simulink model "ame532Project1_GimbalDynamicsModel_2022b"  (R2022b)
settings: Solver=ode4  StartTime=0.0  StopTime=10  FixedStep=0.01  RelTol=1e-3
model workspace (MAT data in the model file):
  theta : Simulink.Parameter (value not decoded)
values from neighbouring files (symbols this model uses):
  a0_s2 = 0    [AeroData.m]
  a0_s3 = 0    [AeroData.m]
  a0_s4 = 0.05    [AeroData.m]
  a0_s5 = 0.05    [AeroData.m]
  CD0_s2 = 0.01    [AeroData.m]
  CD0_s3 = 0.01    [AeroData.m]
  CD0_s4 = 0.01    [AeroData.m]
  CD0_s5 = 0.01    [AeroData.m]
  CDa_s2 = 1    [AeroData.m]
  CDa_s3 = 1    [AeroData.m]
  CDa_s4 = 1    [AeroData.m]
  CDa_s5 = 1    [AeroData.m]
  CL0_s2 = 0    [AeroData.m]
  CL0_s3 = 0    [AeroData.m]
  CL0_s4 = 0.05    [AeroData.m]
  CL0_s5 = 0.05    [AeroData.m]
  CM0_s2 = 0    [AeroData.m]
  CM0_s3 = 0    [AeroData.m]
  CM0_s4 = -0.05    [AeroData.m]
  CM0_s5 = -0.05    [AeroData.m]
  CMa_s2 = 0    [AeroData.m]
  CMa_s3 = 0    [AeroData.m]
  CMa_s4 = 0    [AeroData.m]
  CMa_s5 = 0    [AeroData.m]
  e_s2 = 0.8    [AeroData.m]
  e_s3 = 0.8    [AeroData.m]
  e_s4 = 0.9    [AeroData.m]
  e_s5 = 0.9    [AeroData.m]
  i_s2 = 0    [AeroData.m]
  i_s3 = 0    [AeroData.m]
  i_s4 = 0.05    [AeroData.m]
  i_s5 = 0.05    [AeroData.m]
  Jxx = 1    [Sim_sixDOFdriverScript.m]
  Jxy = 0.    (= 0)    [Sim_sixDOFdriverScript.m]
  Jxz = 3    [Sim_sixDOFdriverScript.m]
  Jyx = 2    [Sim_sixDOFdriverScript.m]
  Jyy = 2    [Sim_sixDOFdriverScript.m]
  Jyz = 0    [Sim_sixDOFdriverScript.m]
  Jzx = Jxz    (= 3)    [Sim_sixDOFdriverScript.m]
  Jzy = Jyz    (= 0)    [Sim_sixDOFdriverScript.m]
  Jzz = 2    [Sim_sixDOFdriverScript.m]
  LL = 0.8    [Sim_sixDOFdriverScript.m]
  MM = 0.8    [Sim_sixDOFdriverScript.m]
  n_s2 = [0; 0; -1]    [AeroData.m]
  n_s3 = [0; 1; 0]    [AeroData.m]
  n_s4 = [0; 0; -1]    [AeroData.m]
  n_s5 = [0; 0; -1]    [AeroData.m]
  NN = 0.8    [Sim_sixDOFdriverScript.m]
  rEarth = 6378100    [Sim_sixDOFdriverScript.m]
  ro = 1.225    [AeroData.m]
undefined symbols (not defined in the file or in its folder): AR_s2, AR_s3, AR_s4, AR_s5, area_s2, area_s3, area_s4, area_s5, c_s2, c_s3, c_s4, c_s5, earthRadius, elevator_sA, leftaileron_sA, mixMatrixInv, rightaileron_sA, rudder_sA, totMass, x_S2_B_B, x_S3_B_B, x_S4_B_B, x_S5_B_B
libraries: simulink_extras x35, matrix_library x22, aerolibutil x8, aerolibfltsims x4, vrlib x4, aerolibtransform2 x2, sharedtransform x2, simulink x2, slpidlib x1, sharedutil x1
(part 4 of 5)

== matlab function ame532Project1_GimbalDynamicsModel_2022b/Gimbal Aircraft dynamic sim/aeroforce coefficient block/MATLAB Function3 ==
  data: alpha input; CM_0 input; CM_s output; CM_a input
function CM_s = calculate_CM_s(alpha,CM_0,CM_a)

CM_s = zeros(4,1);

for i = 1:4
    CM_s(i) = CM_0(i)+CM_a(i)*alpha(i);
end

== matlab function ame532Project1_GimbalDynamicsModel_2022b/Gimbal Aircraft dynamic sim/aeroforce & moment block/MATLAB Function ==
  data: CL_s input; Lift_s output; totalspeed input; area_s input
function Lift_s = calculate_Lift_s(CL_s,totalspeed,area_s)

Lift_s = zeros(4,1);
rho = 1.225; %kg/m3

for i = 1:4
    Lift_s(i) = CL_s(i)*0.5*rho*(totalspeed^2)*area_s(i);
end

end

== matlab function ame532Project1_GimbalDynamicsModel_2022b/Gimbal Aircraft dynamic sim/aeroforce & moment block/MATLAB Function1 ==
  data: aerosurface_matrix input; area_col output
function area_col = extract_area_col(aerosurface_matrix)

area_col = aerosurface_matrix(:,6);

end

== matlab function ame532Project1_GimbalDynamicsModel_2022b/IMU  Aircraft dynamic sim1/Rotational Kinematics/C_BN ==
  data: roll input; ZYXDCM output; pitch input; yaw input
function ZYXDCM = DCM_from_Euler(roll,pitch,yaw) % sequence is yaw pitch roll
    yaw_matrix = [cos(yaw) sin(yaw) 0;
                  -sin(yaw) cos(yaw) 0;
                  0 0 1];
    pitch_matrix = [cos(pitch) 0 -sin(pitch);
                    0           1           0;
                    sin(pitch) 0  cos(pitch)];
    roll_matrix = [1            0           0;
                    0          cos(roll)    sin(roll);
                    0           -sin(roll)  cos(roll)];
    ZYXDCM = roll_matrix*pitch_matrix*yaw_matrix;
end

== matlab function ame532Project1_GimbalDynamicsModel_2022b/Gimbal Aircraft dynamic sim/aeroforce & moment block/MATLAB Function2 ==
  data: CD_s input; Drag_s output; totalspeed input; area_s input
function Drag_s = calculate_Drag_s(CD_s,totalspeed,area_s)

Drag_s = zeros(4,1);
rho = 1.225; %kg/m3

for i = 1:4
    Drag_s(i) = CD_s(i)*0.5*rho*(totalspeed^2)*area_s(i);
end

end

== matlab function ame532Project1_GimbalDynamicsModel_2022b/Gimbal Aircraft dynamic sim/aeroforce & moment block/MATLAB Function3 ==
  data: CM_s input; Moment_s output; totalspeed input; area_s input; chord_s input
function Moment_s = calculate_Moment_s(CM_s,totalspeed,area_s,chord_s)

Moment_s = zeros(4,1);
rho = 1.225; %kg/m3

for i = 1:4
    Moment_s(i) = CM_s(i)*0.5*rho*(totalspeed^2)*area_s(i)*chord_s(i);
end

end

== matlab function ame532Project1_GimbalDynamicsModel_2022b/Gimbal Aircraft dynamic sim/aeroforce & moment block/MATLAB Function4 ==
  data: aerosurface_matrix input; chord_col output
function chord_col = extract_chord_col(aerosurface_matrix)

chord_col = aerosurface_matrix(:,4);

end

== matlab function ame532Project1_GimbalDynamicsModel_2022b/Gimbal Aircraft dynamic sim/aeroforce & moment block/MATLAB Function5 ==
  data: Lift_s input; F_w_s output; n_vector_s input; Drag_s input
function F_w_s = Calculate_F_w(Lift_s,n_vector_s,Drag_s)

F_w_s = zeros(3,4);

for i = 1:4
    F_w_s(:,i) = Lift_s(i).*n_vector_s(:,i) - [Drag_s(i) 0 0]';
end

== matlab function ame532Project1_GimbalDynamicsModel_2022b/Gimbal Aircraft dynamic sim/aeroforce & moment block/MATLAB Function6 ==
  data: n_vector_s input; M_s input; M_w_s output; F_b_s input; x_b_sb input
function M_w_s = Calculate_M_w(n_vector_s,M_s,F_b_s,x_b_sb)

M_w_s = zeros(3,4);

for i = 1:4
      M_w_s(:,i) = M_s(i)*[0 0 0; 0 0 -1; 0 1 0]*n_vector_s(:,i)+cross(x_b_sb(:,i),F_b_s(:,i));
%     M_w_s(:,i) = M_s(i)*[0 0 0; 0 0 -1; 0 1 0]*n_vector_s(:,i)+cross(F_b_s(:,i),x_b_sb(:,i));

end

== matlab function ame532Project1_GimbalDynamicsModel_2022b/Gimbal Aircraft dynamic sim/mass & aero property calculation/MATLAB Function1 ==
  data: aero_prop_matrix input; m_matrix input; x_b_s_ac output; cg_location input
function x_b_s_ac = calculate_x_b_sb(aero_prop_matrix,m_matrix,cg_location)
%this function calculates vector of each component to CM of aircraft

x_b_sb = zeros(3,4);
x_b_s_ac = zeros(3,4);
for i = 1:4
    x_b_s_ac(:,i) = m_matrix(i,5:7)' + [0.25*aero_prop_matrix(i,4) 0 0]';
    x_b_s_ac(:,i) = x_b_s_ac(:,i)- cg_location;

%     x_b_sb(:,i) = m_matrix(i,5:7)' - cg_location;

end

== matlab function ame532Project1_GimbalDynamicsModel_2022b/Gimbal Aircraft dynamic sim/aeroforce & moment block/MATLAB Function7 ==
  data: forcexyz_w_s_matrix input; force_xyz_w output
function force_xyz_w = sum_all_force_xyz(forcexyz_w_s_matrix)

force_xyz_w = zeros(3,1);

for i = 1:3
    force_xyz_w(i) = sum(forcexyz_w_s_matrix(i,:));
end

== matlab function ame532Project1_GimbalDynamicsModel_2022b/Gimbal Aircraft dynamic sim/aeroforce & moment block/MATLAB Function8 ==
  data: m_b_s input; moments_lmn_b output
function moments_lmn_b = sum_all_moments_b_s(m_b_s)

moments_lmn_b = zeros(3,1);

for i = 1:3
    moments_lmn_b(i) = sum(m_b_s(i,:));
end

== matlab function ame532Project1_GimbalDynamicsModel_2022b/Gimbal Aircraft dynamic sim/aeroforce & moment block/MATLAB Function9 ==
  data: DCM_WB output; v_body_ba input; alpha output; beta output; v_inf output
function [DCM_WB,alpha,beta,v_inf]  = construct_DCM_bw(v_body_ba)

alpha = atan2(v_body_ba(3),v_body_ba(1));
beta = asin(v_body_ba(2)/norm(v_body_ba));

DCM_WB = [cos(beta) sin(beta) 0; -sin(beta) cos(beta) 0; 0 0 1]*[cos(alpha) 0 sin(alpha); 0 1 0; -sin(alpha) 0 cos(alpha)];
v_inf = norm(v_body_ba);
end

== matlab function ame532Project1_GimbalDynamicsModel_2022b/IMU  Aircraft dynamic sim1/Rotational Kinematics/MATLAB Function3 ==
  data: p input; Cross_Product_Matrix output; q input; r input
function Cross_Product_Matrix = omega_to_cross_product_matrix(p,q,r)

    Cross_Product_Matrix =[0 -r q; r 0 -p; -q p 0];

end

== matlab function ame532Project1_GimbalDynamicsModel_2022b/IMU  Aircraft dynamic sim1/Rotational Kinematics/MATLAB Function4 ==
  data: DCM input; roll output; pitch output; yaw output
function [roll, pitch, yaw] = Euler_from_DCM(DCM)
   roll = atan2(DCM(2,3),DCM(3,3));
   pitch = -asin(DCM(1,3));
   yaw = atan2(DCM(1,2),DCM(1,1));
end

== matlab function ame532Project1_GimbalDynamicsModel_2022b/IMU  Aircraft dynamic sim1/Rotational Kinematics/C_EN1 ==
  data: roll input; ZYXDCM output; pitch input; yaw input
function ZYXDCM = DCM_from_Euler(roll,pitch,yaw) % sequence is yaw pitch roll
    yaw_matrix = [cos(yaw) sin(yaw) 0;
                  -sin(yaw) cos(yaw) 0;
                  0 0 1];
    pitch_matrix = [cos(pitch) 0 -sin(pitch);
                    0           1           0;
                    sin(pitch) 0  cos(pitch)];
    roll_matrix = [1            0           0;
                    0          cos(roll)    sin(roll);
                    0           -sin(roll)  cos(roll)];
    ZYXDCM = roll_matrix*pitch_matrix*yaw_matrix;
end

== matlab function ame532Project1_GimbalDynamicsModel_2022b/IMU  Aircraft dynamic sim1/Rotational Kinematics/MATLAB Function5 ==
  data: DCM input; roll output; pitch output; yaw output
function [roll, pitch, yaw] = Euler_from_DCM(DCM)
   roll = atan2(DCM(2,3),DCM(3,3));
   pitch = asin(DCM(1,3));
   yaw = atan2(DCM(1,2),DCM(1,1));
end

== matlab function ame532Project1_GimbalDynamicsModel_2022b/IMU  Aircraft dynamic sim1/Rotational Kinematics/MATLAB Function6 ==
  data: DCM input; roll output; pitch output; yaw output
function [roll, pitch, yaw] = Euler_from_DCM(DCM)
   roll = atan2(DCM(2,3),DCM(3,3));
   pitch = -asin(DCM(1,3));
   yaw = atan2(DCM(1,2),DCM(1,1));
end

== matlab function ame532Project1_GimbalDynamicsModel_2022b/IMU  Aircraft dynamic sim1/Rotational Kinematics/MATLAB Function7 ==
  data: quat input; roll output; pitch output; yaw output
function [roll, pitch, yaw] = Euler_from_Quat(quat)
    DCM = zeros(3,3);
    DCM(1) = (quat(1)^2+quat(2)^2-quat(3)^2-quat(4)^2);
    DCM(2) = 2*(quat(2)*quat(3)-quat(1)*quat(4));
    DCM(3) = 2*(quat(2)*quat(4)+quat(1)*quat(3));
    DCM(4) = 2*(quat(2)*quat(3)+quat(1)*quat(4));
    DCM(5) = (quat(1)^2-quat(2)^2+quat(3)^2-quat(4)^2);
    DCM(6) = 2*(quat(3)*quat(4)-quat(1)*quat(2));
    DCM(7) = 2*(quat(2)*quat(4)-quat(1)*quat(3));
    DCM(8) = 2*(quat(3)*quat(4)+quat(1)*quat(2));
    DCM(9) = (quat(1)^2-quat(2)^2-quat(3)^2+quat(4)^2);

    roll = atan2(DCM(2,3),DCM(3,3));
    pitch = -asin(DCM(1,3));
    yaw = atan2(DCM(1,2),DCM(1,1));
end

== matlab function ame532Project1_GimbalDynamicsModel_2022b/IMU  Aircraft dynamic sim1/Rotational Kinematics/MATLAB Function8 ==
  data: roll input; ZYXquat_inv output; pitch input; yaw input; ZYXquat output
function [ZYXquat_inv,ZYXquat] = Quat_from_Euler(roll,pitch,yaw)
    q_yaw = zeros(4,1);
    q_yaw(1) = cos(yaw/2);
    q_yaw(2:4,1) = sin(yaw/2)*[0 0 1]';

    q_pitch = zeros(4,1);
    q_pitch(1) = cos(pitch/2);
    q_pitch(2:4,1) = sin(pitch/2)*[0 1 0]';

    q_roll = zeros(4,1);
    q_roll(1) = cos(roll/2);
    q_roll(2:4,1) = sin(roll/2)*[1 0 0]';
    
    inv_q_yaw = [q_yaw(1);-q_yaw(2:4)];
    inv_q_pitch = [q_pitch(1);-q_pitch(2:4)];
    inv_q_roll = [q_roll(1);-q_roll(2:4)];

    ZYXquat_inv = quat_mult(quat_mult(inv_q_roll,inv_q_pitch),inv_q_yaw);
    ZYXquat = quat_mult(quat_mult(q_yaw,q_pitch),q_roll);

end

function quat = quat_mult(q1,q2)
    quat = zeros(4,1);
    quat(1) = q1(1)*q2(1)-q1(2)*q2(2)-q1(3)*q2(3)-q1(4)*q2(4);
    quat(2) = q1(1)*q2(2)+q1(2)*q2(1)+q1(3)*q2(4)-q1(4)*q2(3);
    quat(3) = q1(1)*q2(3)-q1(2)*q2(4)+q1(3)*q2(1)+q1(4)*q2(2);
    quat(4) = q1(1)*q2(4)+q1(2)*q2(3)-q1(3)*q2(2)+q1(4)*q2(1);
end

== matlab function ame532Project1_GimbalDynamicsModel_2022b/IMU  Aircraft dynamic sim1/Rotational Kinematics/MATLAB Function9 ==
  data: q1 input; quat output; q2 input
function quat = quat_mult(q1,q2)
    quat = zeros(4,1);
    quat(1) = q1(1)*q2(1)-q1(2)*q2(2)-q1(3)*q2(3)-q1(4)*q2(4);
    quat(2) = q1(1)*q2(2)+q1(2)*q2(1)+q1(3)*q2(4)-q1(4)*q2(3);
    quat(3) = q1(1)*q2(3)-q1(2)*q2(4)+q1(3)*q2(1)+q1(4)*q2(2);
    quat(4) = q1(1)*q2(4)+q1(2)*q2(3)-q1(3)*q2(2)+q1(4)*q2(1);
end

== matlab function ame532Project1_GimbalDynamicsModel_2022b/IMU  Aircraft dynamic sim1/Translational Kinematics/C_EN from LAX to ECEF ==
  data: lat input; ZYXDCM output; long input
function ZYXDCM = DCM_from_Euler(lat,long) % sequence of rotation is lat long
%     yaw_matrix = [cos(yaw) sin(yaw) 0;
%                   -sin(yaw) cos(yaw) 0;
%                   0 0 1];
    lat_matrix = [cos(lat) 0 -sin(lat);
                    0           1           0;
                    sin(lat) 0  cos(lat)];
    long_matrix = [1            0           0;
                    0          cos(-long)    sin(-long);
                    0           -sin(-long)  cos(-long)];

    adjust_matrix = [cos(pi/2) 0 -sin(pi/2);
                    0           1           0;
                    sin(pi/2) 0  cos(pi/2)];
    ZYXDCM = adjust_matrix*long_matrix*lat_matrix;
end

%this rotational matrix turns lat long coordinate into a new C_EN
%assuming the N CS is lat and longitudinally rotated, then you would do
%-longditudinal rotation then lat rotation, then rotate 90 degrees again to
%match ECEF

== matlab function ame532Project1_GimbalDynamicsModel_2022b/IMU  Aircraft dynamic sim1/Translational Kinematics/new C_EN base on cart. coordinate1 ==
  data: lat input; ZYXDCM output; long input
function ZYXDCM = DCM_from_Euler(lat,long) % sequence of rotation is lat long
%     yaw_matrix = [cos(yaw) sin(yaw) 0;
%                   -sin(yaw) cos(yaw) 0;
%                   0 0 1];
    lat_matrix = [cos(lat) 0 -sin(lat);
                    0           1           0;
                    sin(lat) 0  cos(lat)];
    long_matrix = [1            0           0;
                    0          cos(-long)    sin(-long);
                    0           -sin(-long)  cos(-long)];

    adjust_matrix = [cos(pi/2) 0 -sin(pi/2);
                    0           1           0;
                    sin(pi/2) 0  cos(pi/2)];
    ZYXDCM = adjust_matrix*long_matrix*lat_matrix;
end

%this rotational matrix turns lat long coordinate into a new C_EN
%assuming the N CS is lat and longitudinally rotated, then you would do
%-longditudinal rotation then lat rotation, then rotate 90 degrees again to
%match ECEF

== matlab function ame532Project1_GimbalDynamicsModel_2022b/IMU  Aircraft dynamic sim1/Unused tranlational kinmatics/C_EN4 ==
  data: roll input; ZYXDCM output; pitch input; yaw input
function ZYXDCM = DCM_from_Euler(roll,pitch,yaw) % sequence is yaw pitch roll
    yaw_matrix = [cos(yaw) sin(yaw) 0;
                  -sin(yaw) cos(yaw) 0;
                  0 0 1];
    pitch_matrix = [cos(pitch) 0 -sin(pitch);
                    0           1           0;
                    sin(pitch) 0  cos(pitch)];
    roll_matrix = [1            0           0;
                    0          cos(roll)    sin(roll);
                    0           -sin(roll)  cos(roll)];
    ZYXDCM = roll_matrix*pitch_matrix*yaw_matrix;
end

== matlab function ame532Project1_GimbalDynamicsModel_2022b/IMU  Aircraft dynamic sim1/aeroforce & moment block/MATLAB Function ==
  data: CL_s input; Lift_s output; totalspeed input; area_s input
function Lift_s = calculate_Lift_s(CL_s,totalspeed,area_s)

Lift_s = zeros(4,1);
rho = 1.225; %kg/m3

for i = 1:4
    Lift_s(i) = CL_s(i)*0.5*rho*(totalspeed^2)*area_s(i);
end

end

== matlab function ame532Project1_GimbalDynamicsModel_2022b/IMU  Aircraft dynamic sim1/aeroforce & moment block/MATLAB Function1 ==
  data: aerosurface_matrix input; area_col output
function area_col = extract_area_col(aerosurface_matrix)

area_col = aerosurface_matrix(:,6);

end

== matlab function ame532Project1_GimbalDynamicsModel_2022b/IMU  Aircraft dynamic sim1/Rotational Kinematics/C_EN2 ==
  data: roll input; ZYXDCM output; pitch input; yaw input
function ZYXDCM = DCM_from_Euler(roll,pitch,yaw) % sequence is yaw pitch roll
    yaw_matrix = [cos(yaw) -sin(yaw) 0;
                  sin(yaw) cos(yaw) 0;
                  0 0 1];
    pitch_matrix = [cos(pitch) 0 sin(pitch);
                    0           1           0;
                    -sin(pitch) 0  cos(pitch)];
    roll_matrix = [1            0           0;
                    0          cos(roll)    -sin(roll);
                    0           sin(roll)  cos(roll)];
    ZYXDCM = roll_matrix*pitch_matrix*yaw_matrix;
end

== matlab function ame532Project1_GimbalDynamicsModel_2022b/IMU  Aircraft dynamic sim1/aeroforce & moment block/MATLAB Function2 ==
  data: CD_s input; Drag_s output; totalspeed input; area_s input
function Drag_s = calculate_Drag_s(CD_s,totalspeed,area_s)

Drag_s = zeros(4,1);
rho = 1.225; %kg/m3

for i = 1:4
    Drag_s(i) = CD_s(i)*0.5*rho*(totalspeed^2)*area_s(i);
end

end

== matlab function ame532Project1_GimbalDynamicsModel_2022b/IMU  Aircraft dynamic sim1/aeroforce & moment block/MATLAB Function3 ==
  data: CM_s input; Moment_s output; totalspeed input; area_s input; chord_s input
function Moment_s = calculate_Moment_s(CM_s,totalspeed,area_s,chord_s)

Moment_s = zeros(4,1);
rho = 1.225; %kg/m3

for i = 1:4
    Moment_s(i) = CM_s(i)*0.5*rho*(totalspeed^2)*area_s(i)*chord_s(i);
end

end

== matlab function ame532Project1_GimbalDynamicsModel_2022b/IMU  Aircraft dynamic sim1/aeroforce & moment block/MATLAB Function4 ==
  data: aerosurface_matrix input; chord_col output
function chord_col = extract_chord_col(aerosurface_matrix)

chord_col = aerosurface_matrix(:,4);

end

== matlab function ame532Project1_GimbalDynamicsModel_2022b/IMU  Aircraft dynamic sim1/aeroforce & moment block/MATLAB Function5 ==
  data: Lift_s input; F_w_s output; n_vector_s input; Drag_s input
function F_w_s = Calculate_F_w(Lift_s,n_vector_s,Drag_s)

F_w_s = zeros(3,4);

for i = 1:4
    F_w_s(:,i) = Lift_s(i).*n_vector_s(:,i) - [Drag_s(i) 0 0]';
end

== matlab function ame532Project1_GimbalDynamicsModel_2022b/IMU  Aircraft dynamic sim1/aeroforce & moment block/MATLAB Function6 ==
  data: n_vector_s input; M_s input; M_w_s output; F_b_s input; x_b_sb input
function M_w_s = Calculate_M_w(n_vector_s,M_s,F_b_s,x_b_sb)

M_w_s = zeros(3,4);

for i = 1:4
      M_w_s(:,i) = M_s(i)*[0 0 0; 0 0 -1; 0 1 0]*n_vector_s(:,i)+cross(x_b_sb(:,i),F_b_s(:,i));
%     M_w_s(:,i) = M_s(i)*[0 0 0; 0 0 -1; 0 1 0]*n_vector_s(:,i)+cross(F_b_s(:,i),x_b_sb(:,i));

end

== matlab function ame532Project1_GimbalDynamicsModel_2022b/IMU  Aircraft dynamic sim1/aeroforce & moment block/MATLAB Function7 ==
  data: forcexyz_w_s_matrix input; force_xyz_w output
function force_xyz_w = sum_all_force_xyz(forcexyz_w_s_matrix)

force_xyz_w = zeros(3,1);

for i = 1:3
    force_xyz_w(i) = sum(forcexyz_w_s_matrix(i,:));
end

== matlab function ame532Project1_GimbalDynamicsModel_2022b/IMU  Aircraft dynamic sim1/aeroforce & moment block/MATLAB Function8 ==
  data: m_b_s input; moments_lmn_b output
function moments_lmn_b = sum_all_moments_b_s(m_b_s)

moments_lmn_b = zeros(3,1);

for i = 1:3
    moments_lmn_b(i) = sum(m_b_s(i,:));
end

== matlab function ame532Project1_GimbalDynamicsModel_2022b/IMU  Aircraft dynamic sim1/aeroforce & moment block/MATLAB Function9 ==
  data: DCM_WB output; v_body_ba input; alpha output; beta output; v_inf output
function [DCM_WB,alpha,beta,v_inf]  = construct_DCM_bw(v_body_ba)

alpha = atan2(v_body_ba(3),v_body_ba(1));
beta = asin(v_body_ba(2)/norm(v_body_ba));

DCM_WB = [cos(beta) sin(beta) 0; -sin(beta) cos(beta) 0; 0 0 1]*[cos(alpha) 0 sin(alpha); 0 1 0; -sin(alpha) 0 cos(alpha)];
v_inf = norm(v_body_ba);
end

== matlab function ame532Project1_GimbalDynamicsModel_2022b/IMU  Aircraft dynamic sim1/aeroforce coefficient block/MATLAB Function ==
  data: AR_matrix input; CL_a output
function CL_a = Calculate_CL_a(AR_matrix)

CL_a = zeros(4,1);

for i = 1:4
    CL_a(i) = 2*pi*(AR_matrix(i)/(2+AR_matrix(i)));
end

== matlab function ame532Project1_GimbalDynamicsModel_2022b/IMU  Aircraft dynamic sim1/aeroforce coefficient block/MATLAB Function1 ==
  data: CL0 input; CL_s output; CL_a input; alpha input
function CL_s = calculate_CL_s(CL0,CL_a,alpha)

CL_s = zeros(4,1);

for i = 1:4
    CL_s(i) = CL0(i)+CL_a(i)*alpha(i);
end

== matlab function ame532Project1_GimbalDynamicsModel_2022b/IMU  Aircraft dynamic sim1/aeroforce coefficient block/MATLAB Function2 ==
  data: CD_0 input; CD_a input; CD_s output; alpha_0 input; alpha input; CL_s input; e input; AR input
function CD_s = calculate_CD_s(CD_0,CD_a,alpha_0,alpha,CL_s,e,AR)
CD_s = zeros(4,1);

for i = 1:4
    
    CD_s(i) = CD_0(i) + CD_a(i)*(alpha(i)-alpha_0(i))^2+(CL_s(i)^2)/(pi*e(i)*AR(i));

end

== matlab function ame532Project1_GimbalDynamicsModel_2022b/IMU  Aircraft dynamic sim1/Rotational Kinematics/MATLAB Function2 ==
  data: phi input; H_matrix_inv output; theta input; psi input
function H_matrix_inv = inv_h_matrix_from_euler(phi,theta,psi)

H_matrix_inv = [1, tan(theta)*sin(phi), tan(theta)*cos(phi);
                0,      cos(phi),           -sin(phi);      
                0,     sin(phi)/cos(theta),   cos(phi)/cos(theta)];

end

== matlab function ame532Project1_GimbalDynamicsModel_2022b/IMU  Aircraft dynamic sim1/aeroforce coefficient block/MATLAB Function3 ==
  data: alpha input; CM_0 input; CM_s output; CM_a input
function CM_s = calculate_CM_s(alpha,CM_0,CM_a)

CM_s = zeros(4,1);

for i = 1:4
    CM_s(i) = CM_0(i)+CM_a(i)*alpha(i);
end

== matlab function ame532Project1_GimbalDynamicsModel_2022b/IMU  Aircraft dynamic sim1/aeroforce coefficient block/calculatie alpha ==
  data: i0 input; alpha output; v_B input; n_vector input; wind_w input; v_B_BA output; C_BN input
function [alpha,v_B_BA] = fcn(i0,v_B,n_vector,wind_w,C_BN)

alpha = zeros(4,1);
% this function calculates alpha that the aero surface sees

v_B_BA = v_B - C_BN*wind_w;

for i = 1:4
    alpha(i) = i0(i) - asin(dot(v_B_BA,n_vector(:,i))/norm(v_B_BA));
end

== matlab function ame532Project1_GimbalDynamicsModel_2022b/IMU  Aircraft dynamic sim1/aeroforce coefficient block/extract matrix function ==
  data: aero_surface_matrix input; AR_matrix output
function AR_matrix = Extract_AR(aero_surface_matrix)

AR_matrix = aero_surface_matrix(:,7);
end

== matlab function ame532Project1_GimbalDynamicsModel_2022b/IMU  Aircraft dynamic sim1/aeroforce coefficient block/extract matrix function1 ==
  data: aero_surface_matrix input; AR_matrix output
function AR_matrix = Extract_AR(aero_surface_matrix)

AR_matrix = aero_surface_matrix(:,7);
end

== matlab function ame532Project1_GimbalDynamicsModel_2022b/IMU  Aircraft dynamic sim1/mass & aero property calculation/CG calculation ==
  data: M_matrix input; cg_x output; cg_y output; cg_z output
function [cg_x, cg_y, cg_z] = CG_calc(M_matrix)

mass_col = M_matrix(:,1);
x_col = M_matrix(:,5);
y_col = M_matrix(:,6);
z_col = M_matrix(:,7);

cg_x = sum(mass_col.*x_col)/(sum(mass_col));
cg_y = sum(mass_col.*y_col)/(sum(mass_col));
cg_z = sum(mass_col.*z_col)/(sum(mass_col));

end

== matlab function ame532Project1_GimbalDynamicsModel_2022b/IMU  Aircraft dynamic sim1/mass & aero property calculation/MATLAB Function ==
  data: cg_location input; M_matrix input; J_matrix output
function J_matrix = fcn(cg_location,M_matrix)


mass_col = M_matrix(:,1);
x_dim = M_matrix(:,2);
y_dim = M_matrix(:,3);
z_dim = M_matrix(:,4);
x_loc = M_matrix(:,5);
y_loc = M_matrix(:,6);
z_loc = M_matrix(:,7);

Ixx = zeros(11,1);
Iyy = zeros(11,1);
Izz = zeros(11,1);
Ixz = zeros(11,1);
Izx = Ixz;
Ixy = zeros(11,1);
Iyx = Ixy;
Iyz = zeros(11,1);
Izy = Iyz;

J_matrix = zeros(3,3);

% all moment of inertial is calculated wrt to CG

for i = 1:11
    Ixx(i) = mass_col(i)*(y_dim(i)^2+z_dim(i)^2)/(12)+mass_col(i)*((y_loc(i)-cg_location(2))^2+(z_loc(i)-cg_location(3))^2); % check discussion post
    Iyy(i) = mass_col(i)*(x_dim(i)^2+z_dim(i)^2)/(12)+mass_col(i)*((x_loc(i)-cg_location(1))^2+(z_loc(i)-cg_location(3))^2);
    Izz(i) = mass_col(i)*(y_dim(i)^2+x_dim(i)^2)/(12)+mass_col(i)*((y_loc(i)-cg_location(2))^2+(x_loc(i)-cg_location(1))^2);
    Ixz(i) = mass_col(i)*((z_loc(i)-cg_location(3))*(x_loc(i)-cg_location(1)));
    Ixy(i) = mass_col(i)*((x_loc(i)-cg_location(1))*(y_loc(i)-cg_location(2)));
    Iyz(i) = mass_col(i)*((y_loc(i)-cg_location(2))*(z_loc(i)-cg_location(3)));


end

J_matrix(1,1) = sum(Ixx);
J_matrix(2,2) = sum(Iyy);
J_matrix(3,3) = sum(Izz);
J_matrix(1,2) = sum(Ixy);
J_matrix(2,1) = sum(Ixy);
J_matrix(1,3) = sum(Ixz);
J_matrix(3,1) = sum(Ixz);
J_matrix(2,3) = sum(Iyz);
J_matrix(3,2) = sum(Iyz);

J_matrix = J_matrix./1000;
end

== matlab function ame532Project1_GimbalDynamicsModel_2022b/IMU  Aircraft dynamic sim1/mass & aero property calculation/MATLAB Function1 ==
  data: aero_prop_matrix input; m_matrix input; x_b_s_ac output; cg_location input
function x_b_s_ac = calculate_x_b_sb(aero_prop_matrix,m_matrix,cg_location)
%this function calculates vector of each component to CM of aircraft

x_b_sb = zeros(3,4);
x_b_s_ac = zeros(3,4);
for i = 1:4
    x_b_s_ac(:,i) = m_matrix(i,5:7)' + [0.25*aero_prop_matrix(i,4) 0 0]';
    x_b_s_ac(:,i) = x_b_s_ac(:,i)- cg_location;

%     x_b_sb(:,i) = m_matrix(i,5:7)' - cg_location;

end

== matlab function ame532Project1_GimbalDynamicsModel_2022b/IMU  Aircraft dynamic sim1/mass & aero property calculation/MATLAB Function2 ==
  data: M_matrix input; aero_prop output
function aero_prop = fcn(M_matrix)

aero_prop = zeros(4,7);
for i = 1:4
    aero_prop(i,1:3) = M_matrix(i,5:7);
    aero_prop(i,4) = M_matrix(i,2);
end

%% define span for each surface

    aero_prop(1,5) = M_matrix(1,3); %right wing
    aero_prop(2,5) = M_matrix(2,3); %left wing
    aero_prop(3,5) = M_matrix(3,3); %hor stab.
    aero_prop(4,5) = M_matrix(4,4); %ver stab.
%% define area and aspect ratio for each surface

for i = 1:4
    aero_prop(i,6) = aero_prop(i,4)*aero_prop(i,5);
    aero_prop(i,7) = aero_prop(i,5)/aero_prop(i,4);
end

== matlab function ame532Project1_GimbalDynamicsModel_2022b/IMU  Aircraft dynamic sim1/measurement subsystem/MATLAB Function ==
  data: velocity input; magnitude output
function magnitude = magnitude_from_vector(velocity)

magnitude = sqrt(velocity(1)^2+velocity(2)^2+velocity(3)^2);

end

== matlab function ame532Project1_GimbalDynamicsModel_2022b/IMU  Aircraft dynamic sim1/translational dynamics/MATLAB Function10 ==
  data: p input; Cross_Product_Matrix output; q input; r input
function Cross_Product_Matrix = omega_to_cross_product_matrix(p,q,r)

    Cross_Product_Matrix =[0 -r q; r 0 -p; -q p 0];

end

== matlab function ame532Project1_GimbalDynamicsModel_2022b/Gimbal Aircraft dynamic sim/Rotational Kinematics/MATLAB Function2 ==
  data: phi input; H_matrix_inv output; theta input; psi input
function H_matrix_inv = inv_h_matrix_from_euler(phi,theta,psi)

H_matrix_inv = [1, tan(theta)*sin(phi), tan(theta)*cos(phi);
                0,      cos(phi),           -sin(phi);      
                0,     sin(phi)/cos(theta),   cos(phi)/cos(theta)];

end

== matlab function ame532Project1_GimbalDynamicsModel_2022b/Gimbal system/magnitude ==
  data: x_E_BG input; R output
function R = fcn(x_E_BG)

R = sqrt(x_E_BG(1)^2+x_E_BG(2)^2+x_E_BG(3)^2);

== matlab function ame532Project1_GimbalDynamicsModel_2022b/Gimbal system/MATLAB Function2 ==
  data: phi input; H_matrix_inv output; theta input; psi input
function H_matrix_inv = inv_h_matrix_from_euler(phi,theta,psi)

H_matrix_inv = [1, tan(theta)*sin(phi), tan(theta)*cos(phi);
                0,      cos(phi),           -sin(phi);      
                0,     sin(phi)/cos(theta),   cos(phi)/cos(theta)];

end

== matlab function ame532Project1_GimbalDynamicsModel_2022b/Gimbal system/Rotational Kinematics/C_BN ==
  data: roll input; ZYXDCM output; pitch input; yaw input
function ZYXDCM = DCM_from_Euler(roll,pitch,yaw) % sequence is yaw pitch roll
    yaw_matrix = [cos(yaw) sin(yaw) 0;
                  -sin(yaw) cos(yaw) 0;
                  0 0 1];
    pitch_matrix = [cos(pitch) 0 -sin(pitch);
                    0           1           0;
                    sin(pitch) 0  cos(pitch)];
    roll_matrix = [1            0           0;
                    0          cos(roll)    sin(roll);
                    0           -sin(roll)  cos(roll)];
    ZYXDCM = roll_matrix*pitch_matrix*yaw_matrix;
end

== matlab function ame532Project1_GimbalDynamicsModel_2022b/Gimbal system/Rotational Kinematics/C_EN1 ==
  data: roll input; ZYXDCM output; pitch input; yaw input
function ZYXDCM = DCM_from_Euler(roll,pitch,yaw) % sequence is yaw pitch roll
    yaw_matrix = [cos(yaw) sin(yaw) 0;
                  -sin(yaw) cos(yaw) 0;
                  0 0 1];
    pitch_matrix = [cos(pitch) 0 -sin(pitch);
                    0           1           0;
                    sin(pitch) 0  cos(pitch)];
    roll_matrix = [1            0           0;
                    0          cos(roll)    sin(roll);
                    0           -sin(roll)  cos(roll)];
    ZYXDCM = roll_matrix*pitch_matrix*yaw_matrix;
end

== matlab function ame532Project1_GimbalDynamicsModel_2022b/Gimbal system/Rotational Kinematics/C_EN2 ==
  data: roll input; ZYXDCM output; pitch input; yaw input
function ZYXDCM = DCM_from_Euler(roll,pitch,yaw) % sequence is yaw pitch roll
    yaw_matrix = [cos(yaw) -sin(yaw) 0;
                  sin(yaw) cos(yaw) 0;
                  0 0 1];
    pitch_matrix = [cos(pitch) 0 sin(pitch);
                    0           1           0;
                    -sin(pitch) 0  cos(pitch)];
    roll_matrix = [1            0           0;
                    0          cos(roll)    -sin(roll);
                    0           sin(roll)  cos(roll)];
    ZYXDCM = roll_matrix*pitch_matrix*yaw_matrix;
end

== matlab function ame532Project1_GimbalDynamicsModel_2022b/Gimbal system/Rotational Kinematics/MATLAB Function2 ==
  data: phi input; H_matrix_inv output; theta input; psi input
function H_matrix_inv = inv_h_matrix_from_euler(phi,theta,psi)

H_matrix_inv = [1, tan(theta)*sin(phi), tan(theta)*cos(phi);
                0,      cos(phi),           -sin(phi);      
                0,     sin(phi)/cos(theta),   cos(phi)/cos(theta)];

end

== matlab function ame532Project1_GimbalDynamicsModel_2022b/Gimbal system/Rotational Kinematics/MATLAB Function3 ==
  data: p input; Cross_Product_Matrix output; q input; r input
function Cross_Product_Matrix = omega_to_cross_product_matrix(p,q,r)

    Cross_Product_Matrix =[0 -r q; r 0 -p; -q p 0];

end

== matlab function ame532Project1_GimbalDynamicsModel_2022b/Gimbal system/Rotational Kinematics/MATLAB Function4 ==
  data: DCM input; roll output; pitch output; yaw output
function [roll, pitch, yaw] = Euler_from_DCM(DCM)
   roll = atan2(DCM(2,3),DCM(3,3));
   pitch = -asin(DCM(1,3));
   yaw = atan2(DCM(1,2),DCM(1,1));
end

== matlab function ame532Project1_GimbalDynamicsModel_2022b/Gimbal system/Rotational Kinematics/MATLAB Function5 ==
  data: DCM input; roll output; pitch output; yaw output
function [roll, pitch, yaw] = Euler_from_DCM(DCM)
   roll = atan2(DCM(2,3),DCM(3,3));
   pitch = asin(DCM(1,3));
   yaw = atan2(DCM(1,2),DCM(1,1));
end

== matlab function ame532Project1_GimbalDynamicsModel_2022b/Gimbal system/Rotational Kinematics/MATLAB Function6 ==
  data: DCM input; roll output; pitch output; yaw output
function [roll, pitch, yaw] = Euler_from_DCM(DCM)
   roll = atan2(DCM(2,3),DCM(3,3));
   pitch = -asin(DCM(1,3));
   yaw = atan2(DCM(1,2),DCM(1,1));
end

== matlab function ame532Project1_GimbalDynamicsModel_2022b/Gimbal Aircraft dynamic sim/Rotational Kinematics/MATLAB Function3 ==
  data: p input; Cross_Product_Matrix output; q input; r input
function Cross_Product_Matrix = omega_to_cross_product_matrix(p,q,r)

    Cross_Product_Matrix =[0 -r q; r 0 -p; -q p 0];

end

== matlab function ame532Project1_GimbalDynamicsModel_2022b/Gimbal system/Rotational Kinematics/MATLAB Function7 ==
  data: quat input; roll output; pitch output; yaw output
function [roll, pitch, yaw] = Euler_from_Quat(quat)
    DCM = zeros(3,3);
    DCM(1) = (quat(1)^2+quat(2)^2-quat(3)^2-quat(4)^2);
    DCM(2) = 2*(quat(2)*quat(3)-quat(1)*quat(4));
    DCM(3) = 2*(quat(2)*quat(4)+quat(1)*quat(3));
    DCM(4) = 2*(quat(2)*quat(3)+quat(1)*quat(4));
    DCM(5) = (quat(1)^2-quat(2)^2+quat(3)^2-quat(4)^2);
    DCM(6) = 2*(quat(3)*quat(4)-quat(1)*quat(2));
    DCM(7) = 2*(quat(2)*quat(4)-quat(1)*quat(3));
    DCM(8) = 2*(quat(3)*quat(4)+quat(1)*quat(2));
    DCM(9) = (quat(1)^2-quat(2)^2-quat(3)^2+quat(4)^2);

    roll = atan2(DCM(2,3),DCM(3,3));
    pitch = -asin(DCM(1,3));
    yaw = atan2(DCM(1,2),DCM(1,1));
end

== matlab function ame532Project1_GimbalDynamicsModel_2022b/Gimbal system/Rotational Kinematics/MATLAB Function8 ==
  data: roll input; ZYXquat_inv output; pitch input; yaw input; ZYXquat output
function [ZYXquat_inv,ZYXquat] = Quat_from_Euler(roll,pitch,yaw)
    q_yaw = zeros(4,1);
    q_yaw(1) = cos(yaw/2);
    q_yaw(2:4,1) = sin(yaw/2)*[0 0 1]';

    q_pitch = zeros(4,1);
    q_pitch(1) = cos(pitch/2);
    q_pitch(2:4,1) = sin(pitch/2)*[0 1 0]';

    q_roll = zeros(4,1);
    q_roll(1) = cos(roll/2);
    q_roll(2:4,1) = sin(roll/2)*[1 0 0]';
    
    inv_q_yaw = [q_yaw(1);-q_yaw(2:4)];
    inv_q_pitch = [q_pitch(1);-q_pitch(2:4)];
    inv_q_roll = [q_roll(1);-q_roll(2:4)];

    ZYXquat_inv = quat_mult(quat_mult(inv_q_roll,inv_q_pitch),inv_q_yaw);
    ZYXquat = quat_mult(quat_mult(q_yaw,q_pitch),q_roll);

end

function quat = quat_mult(q1,q2)
    quat = zeros(4,1);
    quat(1) = q1(1)*q2(1)-q1(2)*q2(2)-q1(3)*q2(3)-q1(4)*q2(4);
    quat(2) = q1(1)*q2(2)+q1(2)*q2(1)+q1(3)*q2(4)-q1(4)*q2(3);
    quat(3) = q1(1)*q2(3)-q1(2)*q2(4)+q1(3)*q2(1)+q1(4)*q2(2);
    quat(4) = q1(1)*q2(4)+q1(2)*q2(3)-q1(3)*q2(2)+q1(4)*q2(1);
end

== matlab function ame532Project1_GimbalDynamicsModel_2022b/Gimbal system/Rotational Kinematics/MATLAB Function9 ==
  data: q1 input; quat output; q2 input
function quat = quat_mult(q1,q2)
    quat = zeros(4,1);
    quat(1) = q1(1)*q2(1)-q1(2)*q2(2)-q1(3)*q2(3)-q1(4)*q2(4);
    quat(2) = q1(1)*q2(2)+q1(2)*q2(1)+q1(3)*q2(4)-q1(4)*q2(3);
    quat(3) = q1(1)*q2(3)-q1(2)*q2(4)+q1(3)*q2(1)+q1(4)*q2(2);
    quat(4) = q1(1)*q2(4)+q1(2)*q2(3)-q1(3)*q2(2)+q1(4)*q2(1);
end

== matlab function ame532Project1_GimbalDynamicsModel_2022b/Gimbal system/Rotational Kinematics/MATLAB Function ==
  data: theta input; H output
function H = HpitchDCM(theta)

H = [cos(theta) 0 -sin(theta); 0 1 0; sin(theta) 0 cos(theta)];

%H = [0 0 0; 0 1 0; sin(theta) 0 cos(theta)];

end

== matlab function ame532Project1_GimbalDynamicsModel_2022b/Gimbal system/DCM_C_OG ==
  data: roll input; ZYXDCM output; pitch input; yaw input
function ZYXDCM = DCM_from_Euler(roll,pitch,yaw) % sequence is yaw pitch roll
    yaw_matrix = [cos(-yaw) sin(-yaw) 0;
                  -sin(-yaw) cos(-yaw) 0;
                  0 0 1];
    pitch_matrix = [cos(-pitch) 0 -sin(-pitch);
                    0           1           0;
                    sin(-pitch) 0  cos(-pitch)];
    roll_matrix = [1            0           0;
                    0          cos(roll)    sin(roll);
                    0           -sin(roll)  cos(roll)];
    ZYXDCM = pitch_matrix*yaw_matrix;
end

== matlab function ame532Project1_GimbalDynamicsModel_2022b/Subsystem/Equations of Motion/Aero Forces and Moments/F&M Horiz Stab Surface (S2)/Compute Aero Lift and Drag ==
  data: alphaLocal output; v_B_A_B input; liftSurf output; dragSurf output; AR_s2 input; i_s2 input; n_s2 input; CL0_s2 input; CD0_s2 input; CDa_s2 input; a0_s2 input; e_s2 input; ro input; area_s2 input; elevatorControl input; elevatorArea_uControl input
function [alphaLocal, liftSurf, dragSurf] = fcn(v_B_A_B, AR_s2, i_s2, n_s2, CL0_s2, CD0_s2, CDa_s2, a0_s2, e_s2, ro, area_s2, elevatorControl, elevatorArea_uControl)
% Compute the lift and drag forces at the respective surface
% arSurf -> Aspect Ratio of respective surfaace
% ro -> air density (note: varies with altitude)
% v_infSurf -> total airspeed at the surface, i.e. Velocity of body w.r.t Inertial/ECEF as
% measured in body frame (|V_B_E_B|)
% v_B_A_B -> relative airspeed, where it is typically 
% v_B_E_B - c_B_N * v_A_N_N and v_A_N_N is the velocity of air mass w.r.t. NED 
% nSurf_B -> Normal force applied at surface
% eSurf -> Oswald efficiency
% alphaLocal0 -> Minimum drag Angle of Attack
delCLsPerdelMu = 3; % ~ About 3 per radian
v_infSurf = norm(v_B_A_B);
cSurfLocAlpha = 2*pi * (AR_s2/(2+AR_s2)); % Lift coefficient at the respective surface due to the local alpha (Angle of Attack)
alphaLocal = i_s2 - asin(dot(v_B_A_B,n_s2)/norm(v_B_A_B)); % in Radians
%cSurfLift = CL0_s2 + cSurfLocAlpha * alphaLocal; % Lift coefficient of surface. Contains no control deflection
cSurfLift = CL0_s2 + cSurfLocAlpha * alphaLocal + (delCLsPerdelMu)*elevatorControl*(elevatorArea_uControl/area_s2); % Lift coefficient of surface
cSurfDrag = CD0_s2 + CDa_s2 *(alphaLocal - a0_s2)^2 + (cSurfLift^2/(pi*e_s2*AR_s2));

liftSurf = cSurfLift * 0.5 * ro * (v_infSurf^2)*area_s2;
dragSurf = cSurfDrag * 0.5 * ro * (v_infSurf^2)*area_s2;

== matlab function ame532Project1_GimbalDynamicsModel_2022b/Subsystem/Equations of Motion/Aero Forces and Moments/F&M Horiz Stab Surface (S2)/Compute Aero Moment ==
  data: V_B_A_B input; momSurf output; alphaLocal input; CM0_s2 input; CMa_s2 input; ro input; area_s2 input; c_s2 input
function momSurf = fcn(V_B_A_B, alphaLocal, CM0_s2, CMa_s2, ro, area_s2, c_s2)
% Compute the Moment at the respective Surface
% v_infSurf -> total airspeed at the surface, i.e. Velocity of body w.r.t Inertial/ECEF as
% measured in body frame (|V_B_E_B|)
% ro -> air density (note: varies with altitude)
% chordSurf -> Chord of the surface area
% cSurfM0 -> Initial moment coefficient of surface
% cSurfMalpha -> Moment coefficient at the respective surface due to the
% local alpha (Angle of Attack)
v_infSurf = norm(V_B_A_B);
cSurfMom = CM0_s2 + CMa_s2*alphaLocal; % Moment coefficient of surface
momSurf = cSurfMom * 0.5 * ro * (v_infSurf^2)*area_s2 * c_s2;

== matlab function ame532Project1_GimbalDynamicsModel_2022b/Subsystem/Equations of Motion/Aero Forces and Moments/F&M Horiz Stab Surface (S2)/F&M in Body/Force Due to Lift and Drag ==
  data: lift input; forceLiftDragS2_B output; drag input; v_B_A_B input; n_s2 input
function forceLiftDragS2_B = fcn(lift, drag, v_B_A_B, n_s2)

forceLiftDrag_w = lift*n_s2 - [drag; 0; 0];
alpha = atan2(v_B_A_B(3), v_B_A_B(1));
beta = asin(v_B_A_B(2) / norm(v_B_A_B));

c_S_B = [cos(alpha), 0, sin(alpha); 0, 1, 0; -sin(alpha), 0, cos(alpha)] ;
c_W_S = [cos(beta), sin(beta), 0; -sin(beta), cos(beta), 0; 0,0,1];
c_W_B = c_W_S * c_S_B;

forceLiftDragS2_B = c_W_B' * forceLiftDrag_w;

== matlab function ame532Project1_GimbalDynamicsModel_2022b/Gimbal Aircraft dynamic sim/Rotational Kinematics/MATLAB Function4 ==
  data: DCM input; roll output; pitch output; yaw output
function [roll, pitch, yaw] = Euler_from_DCM(DCM)
   roll = atan2(DCM(2,3),DCM(3,3));
   pitch = -asin(DCM(1,3));
   yaw = atan2(DCM(1,2),DCM(1,1));
end

== matlab function ame532Project1_GimbalDynamicsModel_2022b/Subsystem/Equations of Motion/Aero Forces and Moments/F&M Horiz Stab Surface (S2)/F&M in Body/Moment S2 ==
  data: momSurf input; momS2_B output; FliftdragS input; n_s2 input; x_S2_B_B input
function momS2_B = fcn(momSurf, FliftdragS, n_s2, x_S2_B_B)
% Compute the moment at the respective surface
crot = [0,0,0; 0,0,-1; 0,1,0];

momS2_B = momSurf * crot* n_s2 + (cross(x_S2_B_B, FliftdragS));

== matlab function ame532Project1_GimbalDynamicsModel_2022b/Subsystem/Equations of Motion/Aero Forces and Moments/F&M Horiz Stab Surface (S3)/Compute Aero Lift and Drag ==
  data: alphaLocal output; v_B_A_B input; liftSurf output; dragSurf output; AR_s3 input; i_s3 input; n_s3 input; CL0_s3 input; CD0_s3 input; CDa_s3 input; a0_s3 input; e_s3 input; ro input; area_s3 input; rudderControl input; rudderarea_uControl input
function [alphaLocal, liftSurf, dragSurf] = fcn(v_B_A_B, AR_s3, i_s3, n_s3, CL0_s3, CD0_s3, CDa_s3, a0_s3, e_s3, ro, area_s3, rudderControl, rudderarea_uControl)
% Compute the lift and drag forces at the respective surface
% arSurf -> Aspect Ratio of respective surfaace
% ro -> air density (note: varies with altitude)
% v_infSurf -> total airspeed at the surface, i.e. Velocity of body w.r.t Inertial/ECEF as
% measured in body frame (|V_B_E_B|)
% v_B_A_B -> relative airspeed, where it is typically 
% v_B_E_B - c_B_N * v_A_N_N and v_A_N_N is the velocity of air mass w.r.t. NED 
% nSurf_B -> Normal force applied at surface
% eSurf -> Oswald efficiency
% alphaLocal0 -> Minimum drag Angle of Attack
delCLsPerdelMu = 3; % ~ About 3 per radian
v_infSurf = norm(v_B_A_B);
cSurfLocAlpha = 2*pi * (AR_s3/(2+AR_s3)); % Lift coefficient at the respective surface due to the local alpha (Angle of Attack)
alphaLocal = i_s3 - asin(dot(v_B_A_B,n_s3)/norm(v_B_A_B)); % in Radians
%cSurfLift = CL0_s3 + cSurfLocAlpha * alphaLocal; % Lift coefficient of surface
cSurfLift = CL0_s3 + cSurfLocAlpha * alphaLocal + (delCLsPerdelMu)*rudderControl*(rudderarea_uControl/area_s3); % Lift coefficient of surface
cSurfDrag = CD0_s3 + CDa_s3 *(alphaLocal - a0_s3)^2 + (cSurfLift^2/(pi*e_s3*AR_s3));

liftSurf = cSurfLift * 0.5 * ro * (v_infSurf^2)*area_s3;
dragSurf = cSurfDrag * 0.5 * ro * (v_infSurf^2)*area_s3;

== matlab function ame532Project1_GimbalDynamicsModel_2022b/Subsystem/Equations of Motion/Aero Forces and Moments/F&M Horiz Stab Surface (S3)/Compute Aero Moment ==
  data: V_B_A_B input; momSurf output; alphaLocal input; CM0_s3 input; CMa_s3 input; ro input; area_s3 input; c_s3 input
function momSurf = fcn(V_B_A_B, alphaLocal, CM0_s3, CMa_s3, ro, area_s3, c_s3)
% Compute the Moment at the respective Surface
% v_infSurf -> total airspeed at the surface, i.e. Velocity of body w.r.t Inertial/ECEF as
% measured in body frame (|V_B_E_B|)
% ro -> air density (note: varies with altitude)
% chordSurf -> Chord of the surface area
% cSurfM0 -> Initial moment coefficient of surface
% cSurfMalpha -> Moment coefficient at the respective surface due to the
% local alpha (Angle of Attack)
v_infSurf = norm(V_B_A_B);
cSurfMom = CM0_s3 + CMa_s3*alphaLocal; % Moment coefficient of surface
momSurf = cSurfMom * 0.5 * ro * (v_infSurf^2)*area_s3 * c_s3;

== matlab function ame532Project1_GimbalDynamicsModel_2022b/Subsystem/Equations of Motion/Aero Forces and Moments/F&M Horiz Stab Surface (S3)/F&M in Body/Force Due to Lift and Drag ==
  data: lift input; forceLiftDragS3_B output; drag input; v_B_A_B input; n_s3 input
function forceLiftDragS3_B = fcn(lift, drag, v_B_A_B, n_s3)

forceLiftDrag_w = lift*n_s3 - [drag; 0; 0];
alpha = atan2(v_B_A_B(3), v_B_A_B(1));
beta = asin(v_B_A_B(2) / norm(v_B_A_B));

c_S_B = [cos(alpha), 0, sin(alpha); 0, 1, 0; -sin(alpha), 0, cos(alpha)] ;
c_W_S = [cos(beta), sin(beta), 0; -sin(beta), cos(beta), 0; 0,0,1];
c_W_B = c_W_S * c_S_B;

forceLiftDragS3_B = c_W_B' * forceLiftDrag_w;

== matlab function ame532Project1_GimbalDynamicsModel_2022b/Subsystem/Equations of Motion/Aero Forces and Moments/F&M Horiz Stab Surface (S3)/F&M in Body/Moment S3 ==
  data: momSurf input; momS3_B output; FliftdragS input; n_s3 input; x_S3_B_B input
function momS3_B = fcn(momSurf, FliftdragS, n_s3, x_S3_B_B)
% Compute the moment at the respective surface
crot = [0,0,0; 0,0,-1; 0,1,0];

momS3_B = momSurf * crot* n_s3 + (cross(x_S3_B_B, FliftdragS));

== matlab function ame532Project1_GimbalDynamicsModel_2022b/Subsystem/Equations of Motion/Aero Forces and Moments/F&M Right Wing and Servo Surface (S4)/Compute Aero Lift and Drag ==
  data: alphaLocal output; v_B_A_B input; liftSurf output; dragSurf output; AR_s4 input; i_s4 input; n_s4 input; CL0_s4 input; CD0_s4 input; CDa_s4 input; a0_s4 input; e_s4 input; ro input; area_s4 input; rightAileronControl input; rightaileronArea_uControl input
function [alphaLocal, liftSurf, dragSurf] = fcn(v_B_A_B, AR_s4, i_s4, n_s4, CL0_s4, CD0_s4, CDa_s4, a0_s4, e_s4, ro, area_s4, rightAileronControl, rightaileronArea_uControl)
% Compute the lift and drag forces at the respective surface
% arSurf -> Aspect Ratio of respective surfaace
% ro -> air density (note: varies with altitude)
% v_infSurf -> total airspeed at the surface, i.e. Velocity of body w.r.t Inertial/ECEF as
% measured in body frame (|V_B_E_B|)
% v_B_A_B -> relative airspeed, where it is typically 
% v_B_E_B - c_B_N * v_A_N_N and v_A_N_N is the velocity of air mass w.r.t. NED 
% nSurf_B -> Normal force applied at surface
% eSurf -> Oswald efficiency
% alphaLocal0 -> Minimum drag Angle of Attack
delCLsPerdelMu = 3; % ~ About 3 per radian
v_infSurf = norm(v_B_A_B);
cSurfLocAlpha = 2*pi * (AR_s4/(2+AR_s4)); % Lift coefficient at the respective surface due to the local alpha (Angle of Attack)
alphaLocal = i_s4 - asin(dot(v_B_A_B,n_s4)/norm(v_B_A_B)); % in Radians
%cSurfLift = CL0_s4 + cSurfLocAlpha * alphaLocal; % Lift coefficient of surface
cSurfLift = CL0_s4 + cSurfLocAlpha * alphaLocal + (delCLsPerdelMu)*rightAileronControl*(rightaileronArea_uControl/area_s4); % Lift coefficient of surface
cSurfDrag = CD0_s4 + CDa_s4 *(alphaLocal - a0_s4)^2 + (cSurfLift^2/(pi*e_s4*AR_s4));

liftSurf = cSurfLift * 0.5 * ro * (v_infSurf^2)*area_s4;
dragSurf = cSurfDrag * 0.5 * ro * (v_infSurf^2)*area_s4;

== matlab function ame532Project1_GimbalDynamicsModel_2022b/Subsystem/Equations of Motion/Aero Forces and Moments/F&M Right Wing and Servo Surface (S4)/Compute Aero Moment ==
  data: V_B_A_B input; momSurf output; alphaLocal input; CM0_s4 input; CMa_s4 input; ro input; area_s4 input; c_s4 input
function momSurf = fcn(V_B_A_B, alphaLocal, CM0_s4, CMa_s4, ro, area_s4, c_s4)
% Compute the Moment at the respective Surface
% v_infSurf -> total airspeed at the surface, i.e. Velocity of body w.r.t Inertial/ECEF as
% measured in body frame (|V_B_E_B|)
% ro -> air density (note: varies with altitude)
% chordSurf -> Chord of the surface area
% cSurfM0 -> Initial moment coefficient of surface
% cSurfMalpha -> Moment coefficient at the respective surface due to the
% local alpha (Angle of Attack)
v_infSurf = norm(V_B_A_B);
cSurfMom = CM0_s4 + CMa_s4*alphaLocal; % Moment coefficient of surface
momSurf = cSurfMom * 0.5 * ro * (v_infSurf^2)*area_s4 * c_s4;

== matlab function ame532Project1_GimbalDynamicsModel_2022b/Gimbal Aircraft dynamic sim/Rotational Kinematics/C_EN1 ==
  data: roll input; ZYXDCM output; pitch input; yaw input
function ZYXDCM = DCM_from_Euler(roll,pitch,yaw) % sequence is yaw pitch roll
    yaw_matrix = [cos(yaw) sin(yaw) 0;
                  -sin(yaw) cos(yaw) 0;
                  0 0 1];
    pitch_matrix = [cos(pitch) 0 -sin(pitch);
                    0           1           0;
                    sin(pitch) 0  cos(pitch)];
    roll_matrix = [1            0           0;
                    0          cos(roll)    sin(roll);
                    0           -sin(roll)  cos(roll)];
    ZYXDCM = roll_matrix*pitch_matrix*yaw_matrix;
end

== matlab function ame532Project1_GimbalDynamicsModel_2022b/Subsystem/Equations of Motion/Aero Forces and Moments/F&M Right Wing and Servo Surface (S4)/F&M in Body/Force Due to Lift and Drag ==
  data: lift input; forceLiftDragS4_B output; drag input; v_B_A_B input; n_s4 input
function forceLiftDragS4_B = fcn(lift, drag, v_B_A_B, n_s4)

forceLiftDrag_w = lift*n_s4 - [drag; 0; 0];
alpha = atan2(v_B_A_B(3), v_B_A_B(1));
beta = asin(v_B_A_B(2) / norm(v_B_A_B));

c_S_B = [cos(alpha), 0, sin(alpha); 0, 1, 0; -sin(alpha), 0, cos(alpha)] ;
c_W_S = [cos(beta), sin(beta), 0; -sin(beta), cos(beta), 0; 0,0,1];
c_W_B = c_W_S * c_S_B;

forceLiftDragS4_B = c_W_B' * forceLiftDrag_w;

== matlab function ame532Project1_GimbalDynamicsModel_2022b/Subsystem/Equations of Motion/Aero Forces and Moments/F&M Right Wing and Servo Surface (S4)/F&M in Body/Moment S4 ==
  data: momSurf input; momS4_B output; FliftdragS input; n_s4 input; x_S4_B_B input
function momS4_B = fcn(momSurf, FliftdragS, n_s4, x_S4_B_B)
% Compute the moment at the respective surface
crot = [0,0,0; 0,0,-1; 0,1,0];

momS4_B = momSurf * crot* n_s4 + (cross(x_S4_B_B, FliftdragS));
